simulink model "RT_ueb2"  (R2013a)
settings: Solver=ode45  StartTime=0.0  StopTime=10.0  RelTol=1e-3
settings Model: BufferReuse=off  Creator=mainster  LastModifiedBy=mainster
settings OptimizationCC: InlineParams=on  BufferReuse=off
settings DebuggingCC: InitInArrayFormatMsg=none

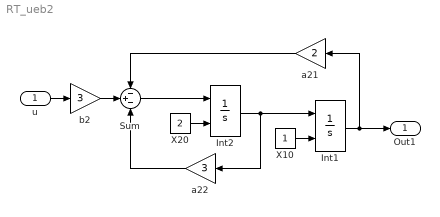
== system RT_ueb2 ==
  u : Inport
  Int1 : Integrator  InitialConditionSource=external  InitialCondition=1
  Int2 : Integrator  InitialConditionSource=external  InitialCondition=2
  Sum : Sum  Inputs=-+-
  X10 : Constant
  X20 : Constant  Value=2
  a21 : Gain  Gain=2
  a22 : Gain  Gain=3
  b2 : Gain  Gain=3
  Out1 : Outport
  wires:
  a21/1 -> Sum/1
  b2/1 -> Sum/2
  Sum/1 -> Int2/1
  a22/1 -> Sum/3
  X20/1 -> Int2/2
  X10/1 -> Int1/2
  u/1 -> b2/1
  Int2/1 -> a22/1, Int1/1
  Int1/1 -> Out1/1, a21/1
